simulink model "controlador_inv_diag"  (R2018b)
settings: Solver=ode23s  StartTime=0.0  StopTime=10  MaxStep=0.05  MinStep=0.0001  RelTol=1e-2
values from neighbouring files (symbols this model uses):
  ref = 0.09    [sliding_mode.m]
  x0 = [0.005; 0; 0.5]    [sliding_mode.m]
undefined symbols (not defined in the file or in its folder): K
settings Model: Creator=User  LastModifiedBy=User

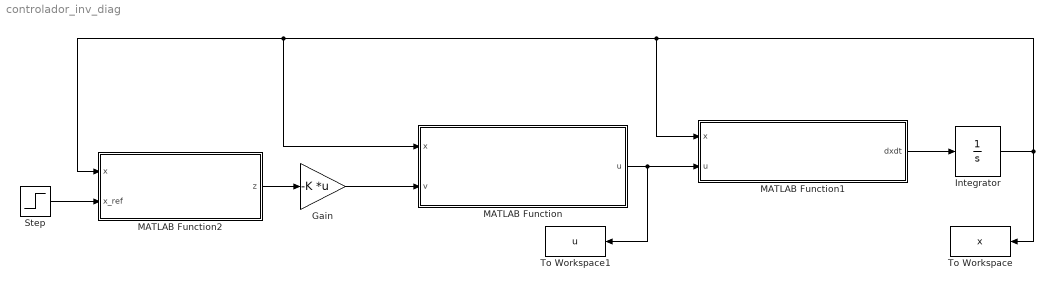
== system controlador_inv_diag ==
  Gain : Gain  Gain=-K  Multiplication=Matrix(K*u)
  Integrator : Integrator  InitialCondition=x0
  MATLAB Function : MATLAB Function  TreatAsAtomicUnit=on
  MATLAB Function1 : MATLAB Function  TreatAsAtomicUnit=on
  MATLAB Function2 : MATLAB Function  TreatAsAtomicUnit=on
  Step : Step  Time=0  After=ref  SampleTime=0
  To Workspace : ToWorkspace  VariableName=x  SaveFormat=Timeseries  SampleTime=-1
  To Workspace1 : ToWorkspace  VariableName=u  SaveFormat=Timeseries  SampleTime=-1
  wires:
  MATLAB Function1/1(dxdt) -> Integrator/1
  MATLAB Function2/1(z) -> Gain/1
  Gain/1 -> MATLAB Function/2(v)
  Integrator/1 -> To Workspace/1, MATLAB Function1/1(x), MATLAB Function/1(x), MATLAB Function2/1(x)
  MATLAB Function/1(u) -> MATLAB Function1/2(u), To Workspace1/1
  Step/1 -> MATLAB Function2/2(x_ref)

== matlab function controlador_inv_diag/MATLAB Function1 ==
  settings: updateMethod=CONTINUOUS  sampleTime=0
  data: x input; u input; dxdt output; paramsr parameter
function dxdt = planta_mls(x, u, paramsr)
    x1 = x(1); x2 = x(2); x3 = x(3);
    params = pn();
    % Troque params por paramsr se quiser adicionar incerteza
    b_nom  = [params.b3, params.b2, params.b1, params.b0];
    Px   = @(y) polyval(b_nom, y);
    
    % Equações de Estado
    dx1 = x2;
    dx2 = params.g - (x3^2)/(params.m * Px(x1));
    dx3 = (1/params.L0) * (u - params.R*x3 - x3*(2/Px(x1))*x2);
    
    dxdt = [dx1; dx2; dx3];
end

== matlab function controlador_inv_diag/MATLAB Function ==
  settings: updateMethod=CONTINUOUS
  data: x input; u output; v input
function u = controlador_inv_dinamica(x, v)
    % x = [posicao; velocidade; corrente]
    % v = sinal do controlador linear
    % params = struct com m, g, R, L0, b0, b1, b2, b3
    params = pn();
    x1 = x(1); x2 = x(2); x3 = x(3);
    b_nom  = [params.b3, params.b2, params.b1, params.b0];
    % Polinômio Denominador e sua derivada
    Px   = @(y) polyval(b_nom, y);
    dPx  = @(y) polyval(polyder(b_nom), y);
    
    % Cálculo de LgLf2h (Ganho de controle)
    LgLf2h = -(2 * x3) / (params.L0 * params.m * Px(x1));
    
    % Cálculo de Lf3h (Dinâmica livre)
    term1 = (2*x3 * (params.R*x3 + (2*x2*x3)/Px(x1))) / (params.L0 * params.m * Px(x1));
    term2 = (x2 * x3^2 * dPx(x1)) / (params.m * Px(x1)^2);
    Lf3h = term1 + term2;
    
    % Lei de Controle por Inversão
    % Adicionado um pequeno valor (1e-6) para evitar divisão por zero se x3=0
    % u = (1 / (LgLf2h - 1e-4 * sign(x3 + 1e-9))) * (-Lf3h + v);
    % Inversão com proteção contra singularidade
    % Se x3 estiver perto de zero, o ganho de controle some.
    % Usamos um limite inferior para LgLf2h
    if abs(LgLf2h) < 1e-4
        Lg_safe = -1e-4; % Mantém o sinal negativo
    else
        Lg_safe = LgLf2h;
    end
    
    u = (1 / Lg_safe) * (-Lf3h + v);
    
    % Saturação física (Tabela I do artigo: 5V)
    if u > 5, u = 5; end
    if u < -5, u = -5; end
end

== matlab function controlador_inv_diag/MATLAB Function2 ==
  settings: updateMethod=CONTINUOUS
  data: x input; z output; x_ref input
function z = coord_transform(x, x_ref)
    % z1 = erro de posição
    % z2 = velocidade (derivada do erro)
    % z3 = aceleração não linear (segunda derivada do erro)
    params = pn();
    x1 = x(1); x2 = x(2); x3 = x(3);
    b_nom  = [params.b3, params.b2, params.b1, params.b0];
    % Polinômio Denominador e sua derivada
    Px   = @(y) polyval(b_nom, y);
    
    z1 = x1 - x_ref;
    z2 = x2;
    z3 = params.g - (x3^2)/(params.m * Px(x1)); % Lf^2 h
    
    z = [z1; z2; z3];
end
